simulink model "model_problem_17"  (R2021a)
settings: Solver=VariableStepAuto  StartTime=0.0  StopTime=8  RelTol=1e-3
model workspace (MAT data in the model file):
  K = 1
values from neighbouring files (symbols this model uses):
  a4 = 0.98    [vars_problem_17_to_21.m]    (also in vars_problem_18_to_21.m; vars_problem_8_to_16.m)
  d1 = 1.5    [vars_problem_17_to_21.m]    (also in vars_problem_18_to_21.m)
  feff = 2.4*10^-5    (= 2.4e-05)    [vars_problem_17_to_21.m]    (also in vars_problem_18_to_21.m; vars_problem_8_to_16.m)
  J_eff = [f(-f_11(x_11)), f(-f_22(x_22)),f(K4),f(2*K1)]    [vars_problem_17_to_21.m]    (also in vars_problem_18_to_21.m; vars_problem_8_to_16.m)
  K_D = [(2*Zeta*w_n*abs(J_eff(1))+1-feff)/kT,(2*Zeta*w_n*abs(J_eff(2))+1-feff)/kT,(2*Zeta*w_n*abs(J_eff(3))+1-feff)/kT,(2*Zeta*w_n*abs(J_eff(4))+1-feff)/kT]    [vars_problem_17_to_21.m]    (also in vars_problem_18_to_21.m; vars_problem_8_to_16.m)
  K_I = [w_n^2/kT,w_n^2/kT,w_n^2/kT,w_n^2/kT]    [vars_problem_17_to_21.m]    (also in vars_problem_18_to_21.m; vars_problem_8_to_16.m)
  K_P = [(2*Zeta*w_n+w_n^2*abs(J_eff(1)))/kT,(2*Zeta*w_n+w_n^2*abs(J_eff(2)))/kT,(2*Zeta*w_n+w_n^2*abs(J_eff(3)))/kT,(2*Zeta*w_n+w_n^2*abs(J_eff(4)))/kT]    [vars_problem_17_to_21.m]    (also in vars_problem_18_to_21.m; vars_problem_8_to_16.m)
  kT = 0.17    [vars_problem_17_to_21.m]    (also in vars_problem_18_to_21.m; vars_problem_8_to_16.m)
  ni = 53    [vars_problem_17_to_21.m]    (also in vars_problem_18_to_21.m; vars_problem_8_to_16.m)
  Tl = [0 fhq_2(q_max) fhq_3(q_max) fhq_4(q_max)]    [vars_problem_17_to_21.m]    (also in vars_problem_18_to_21.m; vars_problem_8_to_16.m)
settings Model: SimulationMode=accelerator  Creator=simon  LastModifiedBy=simon

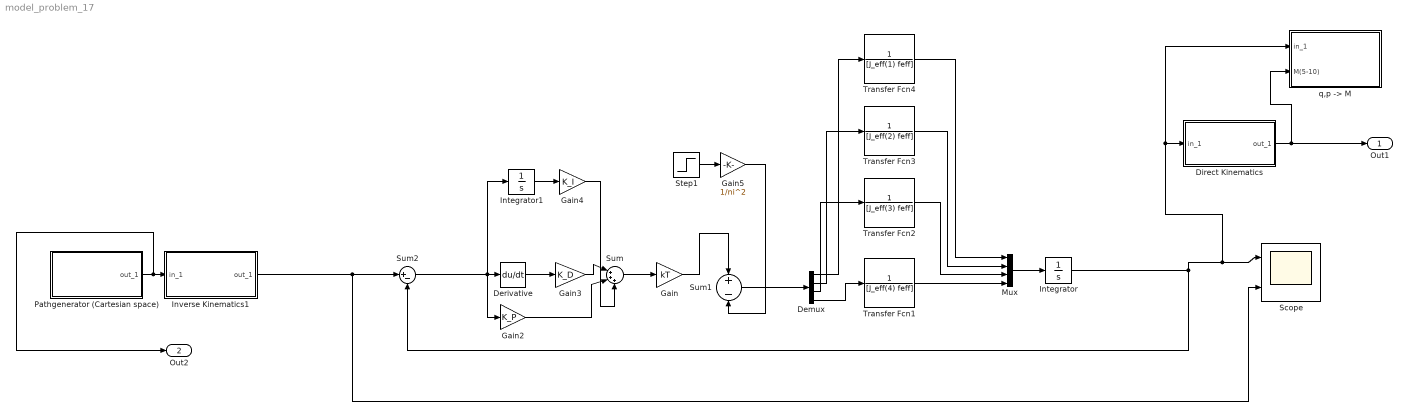
== system model_problem_17 ==
  Demux : Demux
  Derivative : Derivative
  Direct Kinematics : Subsystem
      mask Display: disp('Alto-Robot')
  Gain : Gain  Gain=kT
  Gain2 : Gain  Gain=K_P
  Gain3 : Gain  Gain=K_D
  Gain4 : Gain  Gain=K_I
  Gain5 : Gain  Gain=1/ni^2
  Integrator : Integrator
  Integrator1 : Integrator
  Inverse Kinematics1 : Subsystem
      mask Display: disp('Alto-Robot')
  Mux : Mux
  "Pathgenerator (Cartesian space) " : Subsystem
      mask Display: disp('Alto-Robot\nPath -> p')
  Scope : Scope  NumInputPorts=2
  Step1 : Step  After=Tl  SampleTime=0
  Sum : Sum  Inputs=|+++
  Sum1 : Sum  Inputs=+-
  Sum2 : Sum  Inputs=|+-
  Transfer Fcn1 : TransferFcn  Denominator=[J_eff(4) feff]
  Transfer Fcn2 : TransferFcn  Denominator=[J_eff(3) feff]
  Transfer Fcn3 : TransferFcn  Denominator=[J_eff(2) feff]
  Transfer Fcn4 : TransferFcn  Denominator=[J_eff(1) feff]
  "q,p -> M" : Subsystem
      mask Display: disp('Save to vis4link')
  Out1 : Outport
  Out2 : Outport  Port=2
  wires:
  Integrator/1 -> "q,p -> M"/1(in_1), Direct Kinematics/1(in_1), Scope/1, Sum2/2
  Gain/1 -> Sum1/1
  Inverse Kinematics1/1(out_1) -> Sum2/1, Scope/2
  Sum1/1 -> Demux/1
  Transfer Fcn1/1 -> Mux/4
  Transfer Fcn2/1 -> Mux/3
  Transfer Fcn3/1 -> Mux/2
  Transfer Fcn4/1 -> Mux/1
  Mux/1 -> Integrator/1
  Demux/1 -> Transfer Fcn4/1
  Demux/2 -> Transfer Fcn3/1
  Demux/3 -> Transfer Fcn2/1
  Demux/4 -> Transfer Fcn1/1
  Gain2/1 -> Sum/2
  Sum/1 -> Gain/1
  Sum2/1 -> Integrator1/1, Gain2/1, Derivative/1
  Gain3/1 -> Sum/1
  Derivative/1 -> Gain3/1
  Integrator1/1 -> Gain4/1
  Gain4/1 -> Sum/3
  Step1/1 -> Gain5/1
  Gain5/1 -> Sum1/2
  Direct Kinematics/1(out_1) -> "q,p -> M"/2(M(5-10)), Out1/1
  "Pathgenerator (Cartesian space) "/1(out_1) -> Out2/1, Inverse Kinematics1/1(in_1)

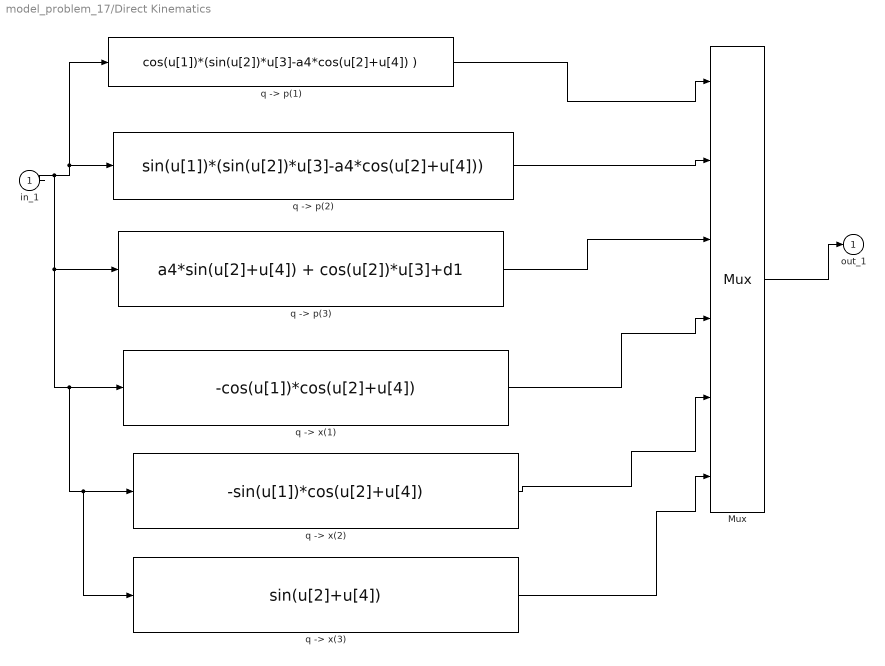
== system model_problem_17/Direct Kinematics ==
  in_1 : Inport
  Mux : Mux  Inputs=6
  "q -> p(1)" : Fcn  Expr=cos(u[1])*(sin(u[2])*u[3]-a4*cos(u[2]+u[4]) )
  "q -> p(2)" : Fcn  Expr=sin(u[1])*(sin(u[2])*u[3]-a4*cos(u[2]+u[4]))
  "q -> p(3)" : Fcn  Expr=a4*sin(u[2]+u[4]) + cos(u[2])*u[3]+d1
  "q -> x(1)" : Fcn  Expr=-cos(u[1])*cos(u[2]+u[4])
  "q -> x(2)" : Fcn  Expr=-sin(u[1])*cos(u[2]+u[4])
  "q -> x(3)" : Fcn  Expr=sin(u[2]+u[4])
  out_1 : Outport  InitialOutput=0  VectorParamsAs1DForOutWhenUnconnected=off
  wires:
  Mux/1 -> out_1/1
  in_1/1 -> "q -> x(3)"/1, "q -> x(2)"/1, "q -> x(1)"/1, "q -> p(3)"/1, "q -> p(2)"/1, "q -> p(1)"/1
  "q -> x(3)"/1 -> Mux/6
  "q -> x(2)"/1 -> Mux/5
  "q -> x(1)"/1 -> Mux/4
  "q -> p(1)"/1 -> Mux/1
  "q -> p(2)"/1 -> Mux/2
  "q -> p(3)"/1 -> Mux/3

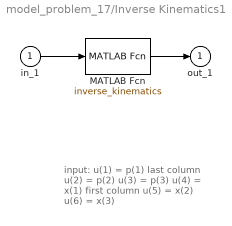
== system model_problem_17/Inverse Kinematics1 ==
  note: input:
      | u(1) = p(1) last column
      | u(2) = p(2)
      | u(3) = p(3)
      | u(4) = x(1) first column
      | u(5) = x(2)
      | u(6) = x(3)
  in_1 : Inport
  MATLAB Fcn : MATLABFcn  MATLABFcn=inverse_kinematics  OutputDimensions=4
  out_1 : Outport  VectorParamsAs1DForOutWhenUnconnected=off
  wires:
  in_1/1 -> MATLAB Fcn/1
  MATLAB Fcn/1 -> out_1/1

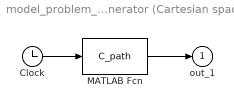
== system model_problem_17/Pathgenerator (Cartesian space)  ==
  Clock : Clock
  MATLAB Fcn : MATLABFcn  MATLABFcn=C_path  OutputDimensions=6
  out_1 : Outport  VectorParamsAs1DForOutWhenUnconnected=off
  wires:
  MATLAB Fcn/1 -> out_1/1
  Clock/1 -> MATLAB Fcn/1

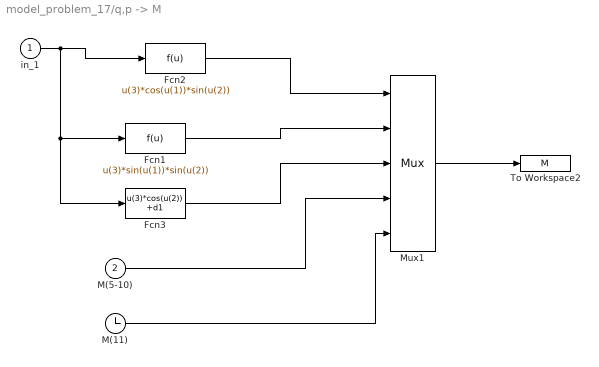
== system model_problem_17/q,p -> M ==
  in_1 : Inport
  M(5-10) : Inport  Port=2
  Fcn1 : Fcn  Expr=u(3)*sin(u(1))*sin(u(2))
  Fcn2 : Fcn  Expr=u(3)*cos(u(1))*sin(u(2))
  Fcn3 : Fcn  Expr=u(3)*cos(u(2)) +d1
  M(11) : Clock
  Mux1 : Mux  Inputs=[1 1 1 6 1]
  To Workspace2 : ToWorkspace  VariableName=M
      settings: MaxDataPoints=100000
  wires:
  Mux1/1 -> To Workspace2/1
  in_1/1 -> Fcn2/1, Fcn1/1, Fcn3/1
  Fcn2/1 -> Mux1/1
  Fcn1/1 -> Mux1/2
  Fcn3/1 -> Mux1/3
  M(5-10)/1 -> Mux1/4
  M(11)/1 -> Mux1/5
